simulink model "EE498_rafetkavak_termproject_part2a_RK_simulinkmodel"  (R2018a)
settings: Solver=ode45  StartTime=0.0  StopTime=10.0  MaxStep=0.001  RelTol=1e-1
values from neighbouring files (symbols this model uses):
  mu = 1/82.45    (= 0.0121285627653)    [EE498_rafetkavak_termproject_part2b_RK_fixedstepsize.m]    (also in EE498_rafetkavak_termproject_part2b_RK_variablestepsize.m)
undefined symbols (not defined in the file or in its folder): mus
libraries: simulink x1
settings Model: Creator=Ersin Keskin  LastModifiedBy=Ersin Keskin

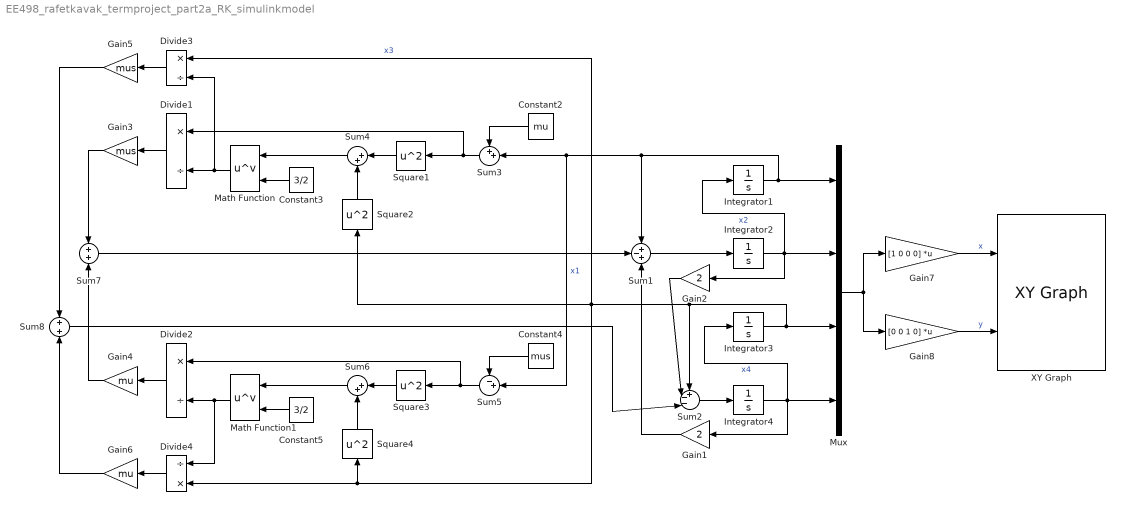
== system EE498_rafetkavak_termproject_part2a_RK_simulinkmodel ==
  Constant2 : Constant  Value=mu
  Constant3 : Constant  Value=3/2
  Constant4 : Constant  Value=mus
  Constant5 : Constant  Value=3/2
  Divide1 : Product  Inputs=*/
  Divide2 : Product  Inputs=*/
  Divide3 : Product  Inputs=*/
  Divide4 : Product  Inputs=/*
  Gain1 : Gain  Gain=2
  Gain2 : Gain  Gain=2
  Gain3 : Gain  Gain=mus
  Gain4 : Gain  Gain=mu
  Gain5 : Gain  Gain=mus
  Gain6 : Gain  Gain=mu
  Gain7 : Gain  Gain=[1 0 0 0]  Multiplication=Matrix(K*u)
  Gain8 : Gain  Gain=[0 0 1 0]  Multiplication=Matrix(K*u)
  Integrator1 : Integrator  InitialCondition=1.2
  Integrator2 : Integrator
  Integrator3 : Integrator
  Integrator4 : Integrator  InitialCondition=-1.0494
  Math Function : Math  Operator=pow  SaturateOnIntegerOverflow=on
  Math Function1 : Math  Operator=pow  SaturateOnIntegerOverflow=on
  Mux : Mux
  Square{1..4} (4 alike) : Math  Operator=square  SaturateOnIntegerOverflow=on
  Sum1 : Sum  Inputs=+-+
  Sum2 : Sum  Inputs=+--|
  Sum3 : Sum  Inputs=++|
  Sum4 : Sum  Inputs=|++
  Sum5 : Sum  Inputs=-+|
  Sum6 : Sum  Inputs=|++
  Sum7 : Sum
  Sum8 : Sum
  XY Graph : simulink/Sinks/XY Graph  xmin=-1.5  xmax=1.5  ymin=-1  ymax=1  st=-1
  wires:
  Math Function1/1 -> Divide2/2, Divide4/1
  Gain5/1 -> Sum8/1
  Divide2/1 -> Gain4/1
  Constant4/1 -> Sum5/1
  Square4/1 -> Sum6/2
  Gain2/1 -> Sum2/2
  Sum1/1 -> Integrator2/1
  Sum2/1 -> Integrator4/1
  Gain3/1 -> Sum7/1
  Sum5/1 -> Square3/1, Divide2/1
  Divide1/1 -> Gain3/1
  Integrator2/1 -> Gain2/1, Integrator1/1, Mux/2  "x2"
  Divide4/1 -> Gain6/1
  Gain4/1 -> Sum7/2
  Integrator4/1 -> Mux/4, Gain1/1, Integrator3/1  "x4"
  Mux/1 -> Gain7/1, Gain8/1
  Sum6/1 -> Math Function1/1
  Integrator1/1 -> Sum5/2, Sum3/2, Sum1/1, Mux/1  "x1"
  Gain6/1 -> Sum8/2
  Sum4/1 -> Math Function/1
  Square1/1 -> Sum4/1
  Constant3/1 -> Math Function/2
  Sum3/1 -> Square1/1, Divide1/1
  Square2/1 -> Sum4/2
  Constant5/1 -> Math Function1/2
  Constant2/1 -> Sum3/1
  Integrator3/1 -> Divide3/1, Divide4/2, Square4/1, Square2/1, Sum2/1, Mux/3  "x3"
  Divide3/1 -> Gain5/1
  Sum7/1 -> Sum1/2
  Gain1/1 -> Sum1/3
  Square3/1 -> Sum6/1
  Math Function/1 -> Divide1/2, Divide3/2
  Sum8/1 -> Sum2/3
  Gain7/1 -> XY Graph/1  "x"
  Gain8/1 -> XY Graph/2  "y"
